simulink model "KalmanSimulimk"  (R2018a)
settings: Solver=VariableStepAuto  StartTime=0.0  StopTime=10.0  RelTol=1e-3
values from neighbouring files (symbols this model uses):
  A = [1 0;     k/m b/m]    [Kalman.m]    (also in fcn.m = [0 1;     -k/m -b/m]; temtProp.m = [0 1;-g/l 0]; untitled2.m = [0 1;     -k/m -b/m])
  B = [0; 1]    [Kalman.m]    (also in fcn.m = [0; 1/m]; temtProp.m = [0;1/(m*l^2)]; untitled2.m = [0; 1/m])
  C = [1 0]    [Kalman.m]    (also in fcn.m = [0 1]; temtProp.m; untitled2.m = [0 1])
  p_pri = A*p_zero*A'    [Kalman.m]    (also in fcn.m = A*p*A + Q)
  x_hzero = [11; 0]    [Kalman.m]    (also in fcn.m = [10; 0]; untitled2.m = [5; 0])
  y = x_zero(1)    [Kalman.m]
settings Model: Creator=Ali  LastModifiedBy=Ali

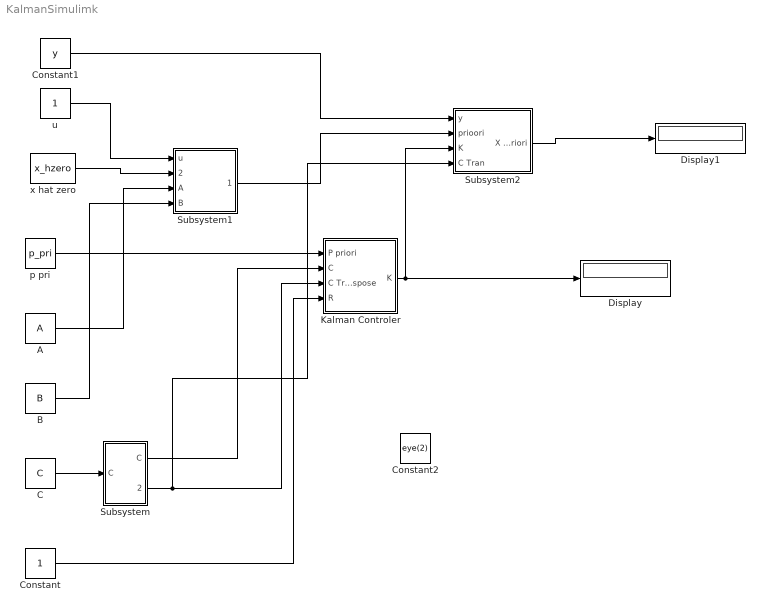
== system KalmanSimulimk ==
  A : Constant  Value=A
  B : Constant  Value=B
  C : Constant  Value=C
  Constant : Constant
  Constant1 : Constant  Value=y
  Constant2 : Constant  Value=eye(2)
  Display : Display
  Display1 : Display
  Kalman Controler : Subsystem
  Subsystem : Subsystem
  Subsystem1 : Subsystem
  Subsystem2 : Subsystem
  p pri : Constant  Value=p_pri
  u : Constant
  x hat zero : Constant  Value=x_hzero
  wires:
  C/1 -> Subsystem/1(C)
  p pri/1 -> Kalman Controler/1(P priori)
  Subsystem/1("C ") -> Kalman Controler/2(C)
  Subsystem/2(C Tran) -> Subsystem2/4(C Tran), Kalman Controler/3(C Transpose)
  Constant/1 -> Kalman Controler/4(R)
  Kalman Controler/1(K) -> Display/1, Subsystem2/3(K)
  u/1 -> Subsystem1/1(u)
  x hat zero/1 -> Subsystem1/2(x hat zero)
  A/1 -> Subsystem1/3(A)
  B/1 -> Subsystem1/4(B)
  Constant1/1 -> Subsystem2/1(y)
  Subsystem1/1(X prioori) -> Subsystem2/2(prioori)
  Subsystem2/1(X posteriori) -> Display1/1

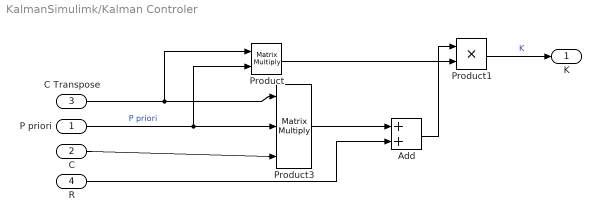
== system KalmanSimulimk/Kalman Controler ==
  P priori : Inport
  C : Inport  Port=2
  C Transpose : Inport  Port=3
  R : Inport  Port=4
  Add : Sum
  Product : Product  Multiplication=Matrix(*)
  Product1 : Product
  Product3 : Product  Inputs=3  Multiplication=Matrix(*)
  K : Outport
  wires:
  C/1 -> Product3/3
  R/1 -> Add/2
  Product3/1 -> Add/1
  Add/1 -> Product1/1
  C Transpose/1 -> Product/1, Product3/1
  Product1/1 -> K/1  "K"
  Product/1 -> Product1/2
  P priori/1 -> Product/2, Product3/2  "P priori"

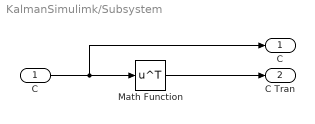
== system KalmanSimulimk/Subsystem ==
  C : Inport
  Math Function : Math  Operator=transpose  SaturateOnIntegerOverflow=on
  "C " : Outport
  C Tran : Outport  Port=2
  wires:
  C/1 -> "C "/1, Math Function/1
  Math Function/1 -> C Tran/1

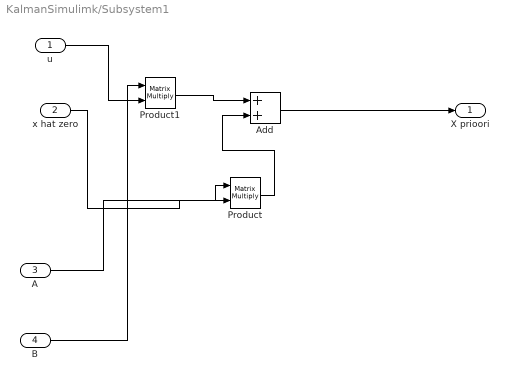
== system KalmanSimulimk/Subsystem1 ==
  u : Inport
  x hat zero : Inport  Port=2
  A : Inport  Port=3
  B : Inport  Port=4
  Add : Sum
  Product : Product  Multiplication=Matrix(*)
  Product1 : Product  Multiplication=Matrix(*)
  X prioori : Outport
  wires:
  A/1 -> Product/1
  Product1/1 -> Add/1
  Add/1 -> X prioori/1
  Product/1 -> Add/2
  u/1 -> Product1/2
  B/1 -> Product1/1
  x hat zero/1 -> Product/2

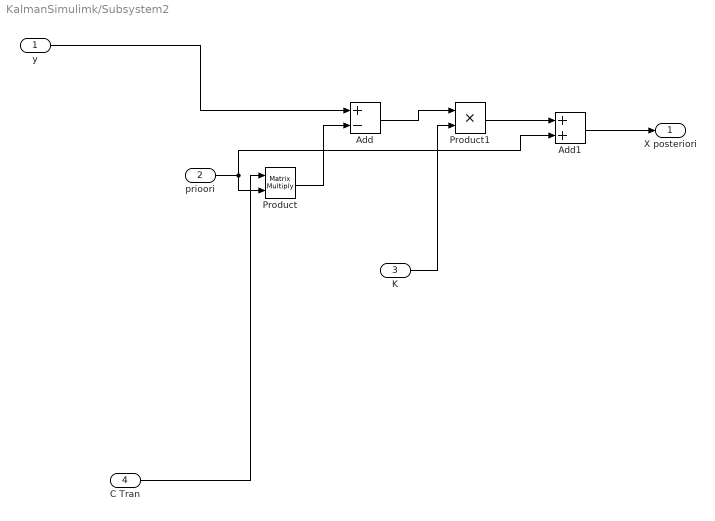
== system KalmanSimulimk/Subsystem2 ==
  y : Inport
  prioori : Inport  Port=2
  K : Inport  Port=3
  C Tran : Inport  Port=4
  Add : Sum  Inputs=+-
  Add1 : Sum
  Product : Product  Multiplication=Matrix(*)
  Product1 : Product
  X posteriori : Outport
  wires:
  Add1/1 -> X posteriori/1
  Add/1 -> Product1/1
  y/1 -> Add/1
  C Tran/1 -> Product/1
  K/1 -> Product1/2
  prioori/1 -> Product/2, Add1/2
  Product/1 -> Add/2
  Product1/1 -> Add1/1
